simulink model "W3Q1"  (R2020b)
settings: Solver=FixedStepDiscrete  StartTime=0.0  StopTime=200  FixedStep=0.1  RelTol=1e-3  EnableMultiTasking=on
settings Model: Creator=VIVEK  LastModifiedBy=VIVEK
settings DataIOCC: LimitDataPoints=on  SaveFormat=Array  ReturnWorkspaceOutputs=off
settings DebuggingCC: SolverPrmCheckMsg=warning  StateNameClashWarn=warning

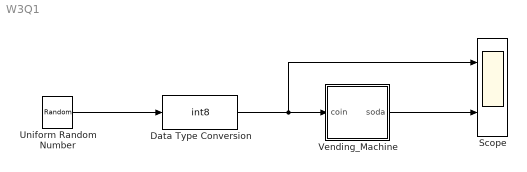
== system W3Q1 ==
  Data Type Conversion : DataTypeConversion  OutDataTypeStr=int8  RndMeth=Nearest  SaturateOnIntegerOverflow=on
  Scope : Scope  NumInputPorts=2
  Uniform Random Number : UniformRandomNumber  Minimum=0  Maximum=2  Seed=500  SampleTime=10
  Vending_Machine : Stateflow chart  TreatAsAtomicUnit=on
  wires:
  Data Type Conversion/1 -> Scope/1, Vending_Machine/1(coin)
  Uniform Random Number/1 -> Data Type Conversion/1
  Vending_Machine/1(soda) -> Scope/2

== stateflow chart W3Q1/Vending_Machine ==
  settings: stateMachineType=MEALY_MACHINE  initializeOutput=1
  state no_coin
  state nickel
  state dime
  (default) -> no_coin
  no_coin -> nickel [order 1] : [coin==1]{soda=0}
  nickel -> no_coin [order 2] : [coin==2]{soda=1}
  dime -> no_coin [order 1] : [coin==1]{soda=1}
  no_coin -> dime [order 2] : [coin==2]{soda=0}
  nickel -> dime [order 1] : [coin==1]{soda=0}
  dime -> nickel [order 2] : [coin==2]{soda=1}
  data: coin input; soda output
